simulink model "Top_Level"  (R2024b)
settings: Solver=ode3  StartTime=0.0  StopTime=1000  RelTol=1e-3  EnableMultiTasking=on
undefined symbols (not defined in the file): dspblkCoreblockFVToolHelper, gcbh, Theta1
libraries: arduinolib x4, arduinosensorlib x3, embeddedblockslib x2
settings Model: ExtModeTrigDuration=2  Creator=muham  LastModifiedBy=muham
settings SolverCC: AlgebraicLoopSolver=TrustRegion  AutoInsertRateTranBlk=on
settings DataIOCC: LimitDataPoints=on  SaveFormat=Array
settings OptimizationCC: ReuseModelBlockBuffer=off  ExpressionDepthLimit=2147483647  LifeSpan=Inf  MaxStackSize=64
settings DebuggingCC: UnderspecifiedInitializationDetection=Classic  MergeDetectMultiDrivingBlocksExec=none  FcnCallInpInsideContextMsg=warning  UnconnectedInputMsg=warning  UnconnectedOutputMsg=warning  UnconnectedLineMsg=warning  AllowSymbolicDim=off  StateNameClashWarn=warning  SFUnexpectedBacktrackingDiag=warning  SFNoUnconditionalDefaultTransitionDiag=warning  SFExecutionAtInitializationDiag=none  ArithmeticOperatorsInVariantConditions=warning
settings HardwareCC: ProdBitPerPointer=32  ProdBitPerSizeT=32  ProdBitPerPtrDiffT=32  ProdLargestAtomicInteger=Long  ProdLargestAtomicFloat=Double  ProdWordSize=32  ProdHWDeviceType=ARM Compatible->ARM Cortex
settings ModelReferenceCC: EnableRefExpFcnMdlSchedulingChecks=on  PropagateSignalLabelsOutOfModel=off
settings SFSimCC: SimUseLocalCustomCode=off  CustomCodeUndefinedFunction=UseInterfaceOnly  SimTargetLang=C++
settings RTWCC: Description=Embedded Coder  SystemTargetFile=ert.tlc  HardwareBoard=ESP32-WROOM(Arduino Compatible)  TemplateMakefile=ert_default_tmf  GenerateReport=on  RTWVerbose=off  RTWUseLocalCustomCode=off  Toolchain=ESP32  BuildConfiguration=Faster Runs  LaunchReport=on  CodeExecutionProfiling=on  GPUComputeCapability=3.5
settings CodeAppCC: ForceParamTrailComments=on  OperatorAnnotations=on  StateflowObjectComments=on  MATLABSourceComments=on
settings ERTTargetCC: TargetLangStandard=C99 (ISO)  MultiwordLength=2048  ERTCustomFileBanners=off  SupportContinuousTime=on  SupportNonInlinedSFcns=on  RemoveResetFunc=off  SupportVariableSizeSignals=on  ModelStepFunctionPrototypeControlCompliant=off  ExtModeTransport=3  ExtModeStaticAlloc=on  ExtModeAutomaticAllocSize=off  ExtModeStaticAllocSize=65536  ExtModeMexFile=ext_xcp  ExtModeIntrfLevel=Level2 - Open  InlinedParameterPlacement=Hierarchical  DynamicArrayContainerType=coder::array
settings ConfigComp: CovMetricSettings=dw  CovSaveCumulativeToWorkspaceVar=on  CovSaveSingleToWorkspaceVar=on  CovExternalEMLEnable=off  CovSFcnEnable=off

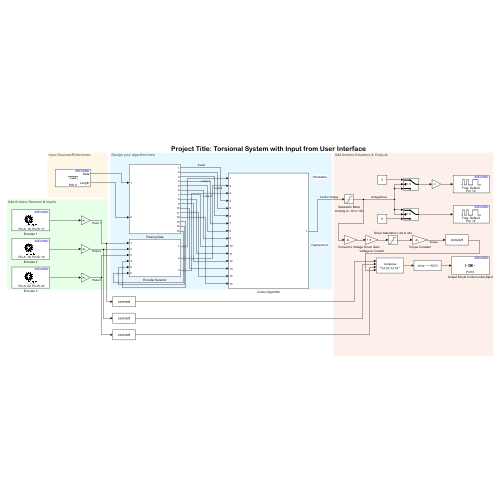
[thumbnail: Simulink's stored preview of the top-level diagram]
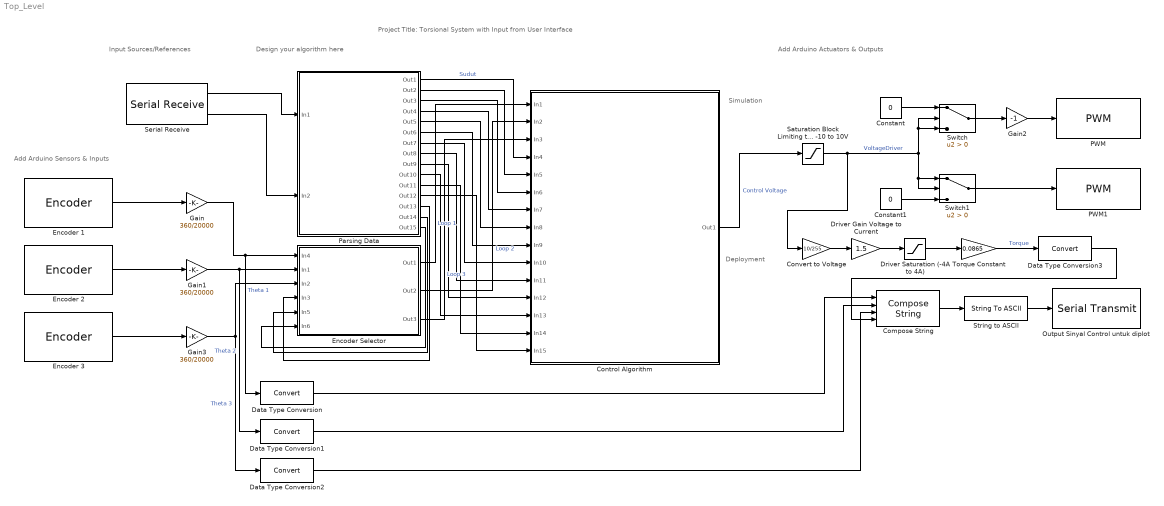
== system Top_Level ==
  note: Deployment
  note: Simulation
  note: Add Arduino Actuators & Outputs
  note: Add Arduino Sensors & Inputs
  note: Design your algorithm here
  note: Input Sources/References
  note: Project Title: Torsional System with Input from User Interface
  Compose String : ComposeString  Format="\"%f,%f,%f,%f\""
  Constant : Constant  Value=0  SampleTime=0.015
  Constant1 : Constant  Value=0  SampleTime=0.015
  Control Algorithm : Subsystem
  Convert to Voltage : Gain  Gain=10/255
  Data Type Conversion{,1..3} (4 alike) : DataTypeConversion  SaturateOnIntegerOverflow=off  RndMeth=Floor
  Driver Gain Voltage to Current : Gain  Gain=1.5
  Driver Saturation (-4A to 4A) : Saturate  UpperLimit=4  LowerLimit=-4
  Encoder 1 : arduinosensorlib/Encoder  InputA=16  InputB=17  Mode=No reset  SampleTime=0.015
  Encoder 2 : arduinosensorlib/Encoder  InputA=18  InputB=19  Mode=No reset  SampleTime=0.015
  Encoder 3 : arduinosensorlib/Encoder  InputA=22  InputB=23  Mode=No reset  SampleTime=0.015
  Encoder Selector : Subsystem
  Gain : Gain  Gain=360/20000
  Gain1 : Gain  Gain=360/20000
  Gain2 : Gain  Gain=-1
  Gain3 : Gain  Gain=360/20000
  Output Sinyal Control untuk diplot : arduinolib/Serial Transmit  portNumber=0  sendmode=write  label=Theta1:  sendformat=Decimal  floatprecision=4  header=uint8('(')  terminator=uint8(')')  blockPlatform=ARDUINO
  PWM : arduinolib/PWM  pinNumber=12  frequencyType=Default  desiredFrequency=490.2  achievableFrequency=490.2
  PWM1 : arduinolib/PWM  pinNumber=14  frequencyType=Default  desiredFrequency=490.2  achievableFrequency=490.2
  Parsing Data : Subsystem
  Saturation Block Limiting to -10 to 10V : Saturate  UpperLimit=255  LowerLimit=-255  OutDataTypeStr=int32
  Serial Receive : arduinolib/Serial Receive  portNumber=0  DataType=uint8  blockPlatform=ARDUINO  TimeOut=0  MaxDataLength=256  isARMArch=off  DataLengthOption=Variable length  Datalength=1  Header=[]  Terminator=[]  SampleTime=0.015  ShowOutStatus=on
  String to ASCII : StringToASCII  OutputVectorSize=48
  Switch : Switch  Criteria=u2 > Threshold  SaturateOnIntegerOverflow=off  InputSameDT=off
  Switch1 : Switch  Criteria=u2 > Threshold  SaturateOnIntegerOverflow=off  InputSameDT=off
  Torque Constant : Gain  Gain=0.0865
  wires:
  Encoder Selector/1(Out1) -> Control Algorithm/1(In1)  "Loop 1"
  Encoder Selector/2(Out2) -> Control Algorithm/2(In2)  "Loop 2"
  Encoder Selector/3(Out3) -> Control Algorithm/3(In3)  "Loop 3"
  Serial Receive/1 -> Parsing Data/1(In1)
  Serial Receive/2 -> Parsing Data/2(In2)
  Parsing Data/1(Out1) -> Control Algorithm/4(In4)  "Sudut"
  Parsing Data/2(Out2) -> Control Algorithm/5(In5)
  Encoder 1/1 -> Gain/1
  Encoder 2/1 -> Gain1/1
  Encoder 3/1 -> Gain3/1
  Parsing Data/13(Out13) -> Encoder Selector/4(In3)
  Parsing Data/14(Out14) -> Encoder Selector/5(In5)
  Parsing Data/15(Out15) -> Encoder Selector/6(In6)
  Parsing Data/3(Out3) -> Control Algorithm/6(In6)
  Parsing Data/4(Out4) -> Control Algorithm/7(In7)
  Parsing Data/5(Out5) -> Control Algorithm/8(In8)
  Parsing Data/6(Out6) -> Control Algorithm/9(In9)
  Parsing Data/7(Out7) -> Control Algorithm/10(In10)
  Parsing Data/8(Out8) -> Control Algorithm/11(In11)
  Parsing Data/9(Out9) -> Control Algorithm/12(In12)
  Parsing Data/10(Out10) -> Control Algorithm/13(In13)
  Parsing Data/11(Out11) -> Control Algorithm/14(In14)
  Parsing Data/12(Out12) -> Control Algorithm/15(In15)
  Saturation Block Limiting to -10 to 10V/1 -> Convert to Voltage/1, Switch1/2, Switch1/1, Switch/2, Switch/3  "VoltageDriver"
  Constant1/1 -> Switch1/3
  Control Algorithm/1(Out1) -> Saturation Block Limiting to -10 to 10V/1  "Control Voltage"
  Gain2/1 -> PWM/1
  Switch/1 -> Gain2/1
  Constant/1 -> Switch/1
  Switch1/1 -> PWM1/1
  Gain/1 -> Data Type Conversion/1, Encoder Selector/1(In4)  "Theta 1"
  Gain1/1 -> Data Type Conversion1/1, Encoder Selector/2(In1)  "Theta 2"
  Gain3/1 -> Data Type Conversion2/1, Encoder Selector/3(In2)  "Theta 3"
  Data Type Conversion/1 -> Compose String/1
  Driver Gain Voltage to Current/1 -> Driver Saturation (-4A to 4A)/1
  Driver Saturation (-4A to 4A)/1 -> Torque Constant/1
  Torque Constant/1 -> Data Type Conversion3/1  "Torque"
  Data Type Conversion1/1 -> Compose String/2
  Data Type Conversion2/1 -> Compose String/3
  Data Type Conversion3/1 -> Compose String/4
  String to ASCII/1 -> Output Sinyal Control untuk diplot/1
  Compose String/1 -> String to ASCII/1
  Convert to Voltage/1 -> Driver Gain Voltage to Current/1

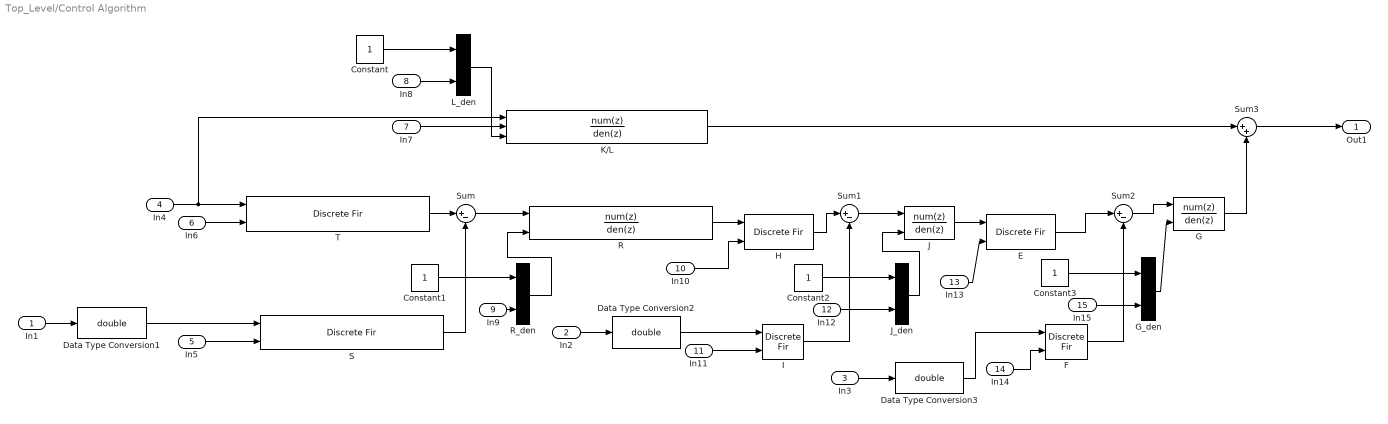
== system Top_Level/Control Algorithm ==
  In1 : Inport
  In2 : Inport  Port=2
  In3 : Inport  Port=3
  In4 : Inport  Port=4
  In5 : Inport  Port=5
  In6 : Inport  Port=6
  In7 : Inport  Port=7
  In8 : Inport  Port=8
  In9 : Inport  Port=9
  In10 : Inport  Port=10
  In11 : Inport  Port=11
  In12 : Inport  Port=12
  In13 : Inport  Port=13
  In14 : Inport  Port=14
  In15 : Inport  Port=15
  Constant{,1..3} (4 alike) : Constant  SampleTime=0.015
  Data Type Conversion1 : DataTypeConversion  OutDataTypeStr=double  SaturateOnIntegerOverflow=off  RndMeth=Floor
  Data Type Conversion2 : DataTypeConversion  OutDataTypeStr=double  SaturateOnIntegerOverflow=off  RndMeth=Floor
  Data Type Conversion3 : DataTypeConversion  OutDataTypeStr=double  SaturateOnIntegerOverflow=off  RndMeth=Floor
  E : DiscreteFir  LoadFcn=dspblkCoreblockFVToolHelper(gcbh,'load');  CoefSource=Input port  Coefficients=[1 1]
      settings: CopyFcn=dspblkCoreblockFVToolHelper(gcbh,'copy');  DeleteFcn=dspblkCoreblockFVToolHelper(gcbh,'close');  ModelCloseFcn=dspblkCoreblockFVToolHelper(gcbh,'close');  PreSaveFcn=dspblkCoreblockFVToolHelper(gcbh,'presave');  PostSaveFcn=dspblkCoreblockFVToolHelper(gcbh,'postsave');  CloseFcn=dspblkCoreblockFVToolHelper(gcbh,'close');  InputPortMap=u0,u1
  F : DiscreteFir  LoadFcn=dspblkCoreblockFVToolHelper(gcbh,'load');  CoefSource=Input port  Coefficients=[1 1]
      settings: CopyFcn=dspblkCoreblockFVToolHelper(gcbh,'copy');  DeleteFcn=dspblkCoreblockFVToolHelper(gcbh,'close');  ModelCloseFcn=dspblkCoreblockFVToolHelper(gcbh,'close');  PreSaveFcn=dspblkCoreblockFVToolHelper(gcbh,'presave');  PostSaveFcn=dspblkCoreblockFVToolHelper(gcbh,'postsave');  CloseFcn=dspblkCoreblockFVToolHelper(gcbh,'close');  InputPortMap=u0,u1
  G : DiscreteFilter  LoadFcn=dspblkCoreblockFVToolHelper(gcbh,'load');  DenominatorSource=Input port  Denominator=[1 1]  a0EqualsOne=on
      settings: CopyFcn=dspblkCoreblockFVToolHelper(gcbh,'copy');  DeleteFcn=dspblkCoreblockFVToolHelper(gcbh,'close');  ModelCloseFcn=dspblkCoreblockFVToolHelper(gcbh,'close');  PreSaveFcn=dspblkCoreblockFVToolHelper(gcbh,'presave');  PostSaveFcn=dspblkCoreblockFVToolHelper(gcbh,'postsave');  CloseFcn=dspblkCoreblockFVToolHelper(gcbh,'close');  InputPortMap=u0,p3
  G_den : Mux  Inputs=2
  H : DiscreteFir  LoadFcn=dspblkCoreblockFVToolHelper(gcbh,'load');  CoefSource=Input port  Coefficients=[1 1]
      settings: CopyFcn=dspblkCoreblockFVToolHelper(gcbh,'copy');  DeleteFcn=dspblkCoreblockFVToolHelper(gcbh,'close');  ModelCloseFcn=dspblkCoreblockFVToolHelper(gcbh,'close');  PreSaveFcn=dspblkCoreblockFVToolHelper(gcbh,'presave');  PostSaveFcn=dspblkCoreblockFVToolHelper(gcbh,'postsave');  CloseFcn=dspblkCoreblockFVToolHelper(gcbh,'close');  InputPortMap=u0,u1
  I : DiscreteFir  LoadFcn=dspblkCoreblockFVToolHelper(gcbh,'load');  CoefSource=Input port  Coefficients=[1 1]
      settings: CopyFcn=dspblkCoreblockFVToolHelper(gcbh,'copy');  DeleteFcn=dspblkCoreblockFVToolHelper(gcbh,'close');  ModelCloseFcn=dspblkCoreblockFVToolHelper(gcbh,'close');  PreSaveFcn=dspblkCoreblockFVToolHelper(gcbh,'presave');  PostSaveFcn=dspblkCoreblockFVToolHelper(gcbh,'postsave');  CloseFcn=dspblkCoreblockFVToolHelper(gcbh,'close');  InputPortMap=u0,u1
  J : DiscreteFilter  LoadFcn=dspblkCoreblockFVToolHelper(gcbh,'load');  DenominatorSource=Input port  Denominator=[1 1]  a0EqualsOne=on
      settings: CopyFcn=dspblkCoreblockFVToolHelper(gcbh,'copy');  DeleteFcn=dspblkCoreblockFVToolHelper(gcbh,'close');  ModelCloseFcn=dspblkCoreblockFVToolHelper(gcbh,'close');  PreSaveFcn=dspblkCoreblockFVToolHelper(gcbh,'presave');  PostSaveFcn=dspblkCoreblockFVToolHelper(gcbh,'postsave');  CloseFcn=dspblkCoreblockFVToolHelper(gcbh,'close');  InputPortMap=u0,p3
  J_den : Mux  Inputs=2
  K/L : DiscreteFilter  LoadFcn=dspblkCoreblockFVToolHelper(gcbh,'load');  NumeratorSource=Input port  Numerator=[1 1 1 1 1 1 1 1]  DenominatorSource=Input port  Denominator=[1 1 1 1 1 1 1 1]  a0EqualsOne=on
      settings: CopyFcn=dspblkCoreblockFVToolHelper(gcbh,'copy');  DeleteFcn=dspblkCoreblockFVToolHelper(gcbh,'close');  ModelCloseFcn=dspblkCoreblockFVToolHelper(gcbh,'close');  PreSaveFcn=dspblkCoreblockFVToolHelper(gcbh,'presave');  PostSaveFcn=dspblkCoreblockFVToolHelper(gcbh,'postsave');  CloseFcn=dspblkCoreblockFVToolHelper(gcbh,'close');  InputPortMap=u0,p1,p3
  L_den : Mux  Inputs=2
  R : DiscreteFilter  LoadFcn=dspblkCoreblockFVToolHelper(gcbh,'load');  DenominatorSource=Input port  Denominator=[1 1 1 1 1 1 1 1]  a0EqualsOne=on
      settings: CopyFcn=dspblkCoreblockFVToolHelper(gcbh,'copy');  DeleteFcn=dspblkCoreblockFVToolHelper(gcbh,'close');  ModelCloseFcn=dspblkCoreblockFVToolHelper(gcbh,'close');  PreSaveFcn=dspblkCoreblockFVToolHelper(gcbh,'presave');  PostSaveFcn=dspblkCoreblockFVToolHelper(gcbh,'postsave');  CloseFcn=dspblkCoreblockFVToolHelper(gcbh,'close');  InputPortMap=u0,p3
  R_den : Mux  Inputs=2
  S : DiscreteFir  LoadFcn=dspblkCoreblockFVToolHelper(gcbh,'load');  CoefSource=Input port  Coefficients=[1 1 1 1 1 1 1 1]
      settings: CopyFcn=dspblkCoreblockFVToolHelper(gcbh,'copy');  DeleteFcn=dspblkCoreblockFVToolHelper(gcbh,'close');  ModelCloseFcn=dspblkCoreblockFVToolHelper(gcbh,'close');  PreSaveFcn=dspblkCoreblockFVToolHelper(gcbh,'presave');  PostSaveFcn=dspblkCoreblockFVToolHelper(gcbh,'postsave');  CloseFcn=dspblkCoreblockFVToolHelper(gcbh,'close');  InputPortMap=u0,u1
  Sum : Sum  Inputs=|+-
  Sum1 : Sum  Inputs=|+-
  Sum2 : Sum  Inputs=|+-
  Sum3 : Sum  Inputs=|++
  T : DiscreteFir  LoadFcn=dspblkCoreblockFVToolHelper(gcbh,'load');  CoefSource=Input port  Coefficients=[1 1 1 1 1 1 1 1]
      settings: CopyFcn=dspblkCoreblockFVToolHelper(gcbh,'copy');  DeleteFcn=dspblkCoreblockFVToolHelper(gcbh,'close');  ModelCloseFcn=dspblkCoreblockFVToolHelper(gcbh,'close');  PreSaveFcn=dspblkCoreblockFVToolHelper(gcbh,'presave');  PostSaveFcn=dspblkCoreblockFVToolHelper(gcbh,'postsave');  CloseFcn=dspblkCoreblockFVToolHelper(gcbh,'close');  InputPortMap=u0,u1
  Out1 : Outport
  wires:
  In1/1 -> Data Type Conversion1/1
  T/1 -> Sum/1
  S/1 -> Sum/2
  Sum/1 -> R/1
  In4/1 -> K/L/1, T/1
  R/1 -> H/1
  In2/1 -> Data Type Conversion2/1
  I/1 -> Sum1/2
  H/1 -> Sum1/1
  Sum1/1 -> J/1
  J/1 -> E/1
  In3/1 -> Data Type Conversion3/1
  E/1 -> Sum2/1
  F/1 -> Sum2/2
  Sum2/1 -> G/1
  K/L/1 -> Sum3/1
  G/1 -> Sum3/2
  In5/1 -> S/2
  In6/1 -> T/2
  In7/1 -> K/L/2
  L_den/1 -> K/L/3
  In8/1 -> L_den/2
  Constant/1 -> L_den/1
  Constant1/1 -> R_den/1
  In9/1 -> R_den/2
  R_den/1 -> R/2
  In10/1 -> H/2
  In11/1 -> I/2
  J_den/1 -> J/2
  Constant2/1 -> J_den/1
  In12/1 -> J_den/2
  In13/1 -> E/2
  In14/1 -> F/2
  Constant3/1 -> G_den/1
  In15/1 -> G_den/2
  G_den/1 -> G/2
  Data Type Conversion1/1 -> S/1
  Data Type Conversion2/1 -> I/1
  Data Type Conversion3/1 -> F/1
  Sum3/1 -> Out1/1

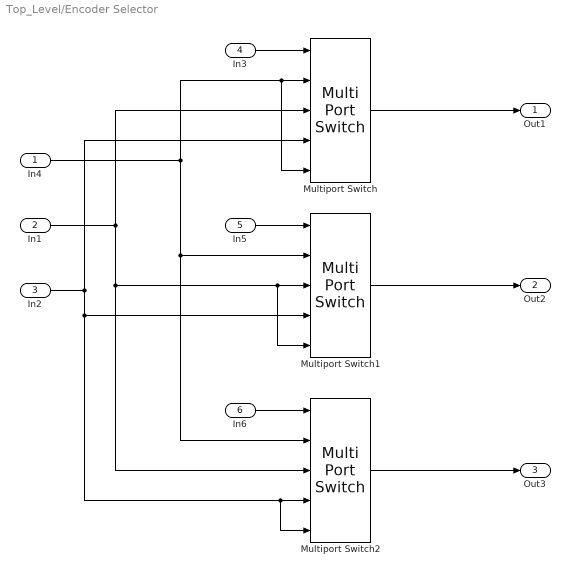
== system Top_Level/Encoder Selector ==
  In4 : Inport
  In1 : Inport  Port=2
  In2 : Inport  Port=3
  In3 : Inport  Port=4
  In5 : Inport  Port=5
  In6 : Inport  Port=6
  Multiport Switch : MultiPortSwitch  DataPortForDefault=Additional data port  DiagnosticForDefault=None  SaturateOnIntegerOverflow=off  InputSameDT=off
  Multiport Switch1 : MultiPortSwitch  DataPortForDefault=Additional data port  DiagnosticForDefault=None  SaturateOnIntegerOverflow=off  InputSameDT=off
  Multiport Switch2 : MultiPortSwitch  DataPortForDefault=Additional data port  DiagnosticForDefault=None  SaturateOnIntegerOverflow=off  InputSameDT=off
  Out1 : Outport
  Out2 : Outport  Port=2
  Out3 : Outport  Port=3
  wires:
  Multiport Switch/1 -> Out1/1
  Multiport Switch1/1 -> Out2/1
  Multiport Switch2/1 -> Out3/1
  In4/1 -> Multiport Switch2/2, Multiport Switch1/2, Multiport Switch/5, Multiport Switch/2
  In1/1 -> Multiport Switch2/3, Multiport Switch1/5, Multiport Switch1/3, Multiport Switch/3
  In2/1 -> Multiport Switch2/5, Multiport Switch2/4, Multiport Switch1/4, Multiport Switch/4
  In3/1 -> Multiport Switch/1
  In5/1 -> Multiport Switch1/1
  In6/1 -> Multiport Switch2/1

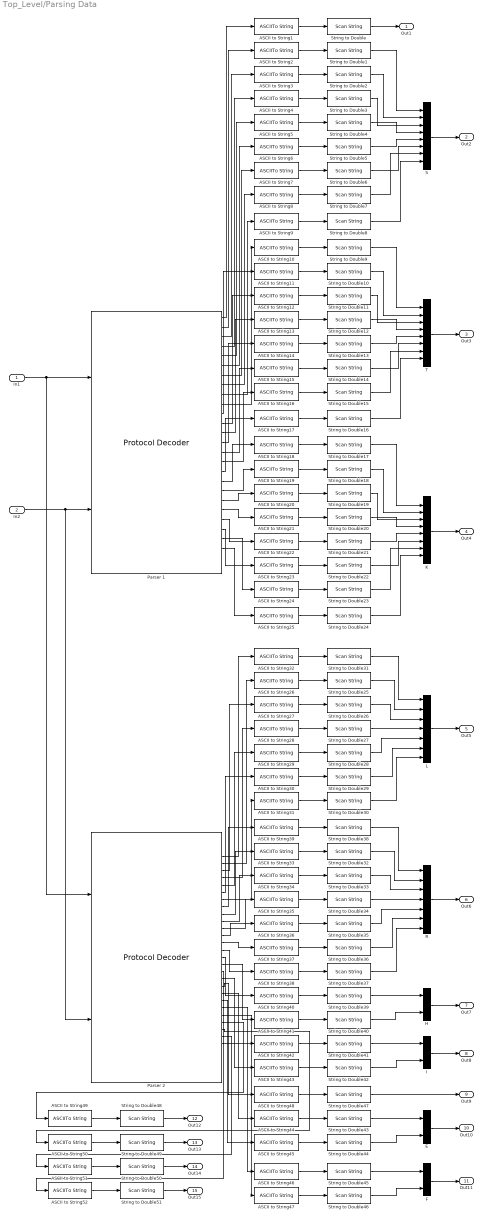
== system Top_Level/Parsing Data ==
  In1 : Inport
  In2 : Inport  Port=2
  ASCII to String{1..52} (52 alike) : ASCIIToString
  E : Mux  Inputs=2
  F : Mux  Inputs=2
  H : Mux  Inputs=2
  I : Mux  Inputs=2
  K : Mux  Inputs=8
  L : Mux  Inputs=7
  Parser 1 : embeddedblockslib/Protocol Decoder  IsParseCSV=on  Header=uint8('#')  FieldTable={ 'Sudut', '4', 'uint8', 'Little endian'; 'S0', '6', 'uint8', 'Little endian'; 'S1', '6', 'uint8', 'Little endian'; 'S2', '6', 'uint8', 'Little endian'; 'S3', '6', 'uint8', 'Little endian'; 'S4', '6', 'uint8', 'Little endian'; 'S5', '6', 'uint8', 'Little endian'; 'S6', '6', 'uint8', 'Little endian'; 'S7', '6', 'uint8', 'Little endian'; 'T0', '6', 'uint8', 'Little endian'; 'T1', '6', 'uint8', 'Little endian'; 'T2', '6', 'uint8', 'Little endian'; 'T3', '6', 'uint8', 'Little endian'; 'T4', '6', 'uint8', 'Little endian'; 'T5', '6', 'uint8', 'Little endian'; 'T6', '6', 'uint8', 'Little endian'; 'T7', '6', 'uint8', 'Little endian'; 'K0', '6', 'uint8', 'Little endian'; 'K1', '6', 'uint8', 'Little endian'; 'K2', '6', 'uint8', 'Little endian'; 'K3', '6', 'uint8', 'Little endian'; 'K4', '6', 'uint8', 'Little endian'; 'K5', '6', 'uint8', 'Little endian'; 'K6', '6', 'uint8', 'Little endian'; 'K7', '6', 'uint8', 'Little endian' }  IsVariableSizeLastField=off  MaxVariableSizeFieldLength=[]  IsChecksumRequired=off  ChecksumAlgorithm=XOR of bytes  ChecksumSize=[]  TerminatorOption=Custom terminator  CustomTerminatorVal=uint8('$')  IsInputLengthAvailable=on  Logo=ARDUINO
      settings: LibrarySourceBlock=arduinolib/Protocol Decoder
  Parser 2 : embeddedblockslib/Protocol Decoder  IsParseCSV=on  Header=uint8('%')  FieldTable={ 'L1', '6', 'uint8', 'Little endian'; 'L2', '6', 'uint8', 'Little endian'; 'L3', '6', 'uint8', 'Little endian'; 'L4', '6', 'uint8', 'Little endian'; 'L5', '6', 'uint8', 'Little endian'; 'L6', '6', 'uint8', 'Little endian'; 'L7', '6', 'uint8', 'Little endian'; 'R1', '6', 'uint8', 'Little endian'; 'R2', '6', 'uint8', 'Little endian'; 'R3', '6', 'uint8', 'Little endian'; 'R4', '6', 'uint8', 'Little endian'; 'R5', '6', 'uint8', 'Little endian'; 'R6', '6', 'uint8', 'Little endian'; 'R7', '6', 'uint8', 'Little endian'; 'H0', '6', 'uint8', 'Little endian'; 'H1', '6', 'uint8', 'Little endian'; 'I0', '6', 'uint8', 'Little endian'; 'I1', '6', 'uint8', 'Little endian'; 'J1', '6', 'uint8', 'Little endian'; 'E0', '6', 'uint8', 'Little endian'; 'E1', '6', 'uint8', 'Little endian'; 'F0', '6', 'uint8', 'Little endian'; 'F1', '6', 'uint8', 'Little endian'; 'G1', '6', 'uint8', 'Little endian'; 'enc1', '1', 'uint8', 'Little endian'; 'enc2', '1', 'uint8', 'Little endian'; 'enc3', '1', 'uint8', 'Little endian' }  IsVariableSizeLastField=off  MaxVariableSizeFieldLength=[]  IsChecksumRequired=off  ChecksumAlgorithm=XOR of bytes  ChecksumSize=[]  TerminatorOption=Custom terminator  CustomTerminatorVal=uint8('^')  IsInputLengthAvailable=on  Logo=ARDUINO
      settings: LibrarySourceBlock=arduinolib/Protocol Decoder
  R : Mux  Inputs=7
  S : Mux  Inputs=8
  String to Double{,1..51} (52 alike) : ScanString  Format="\"%lf\""
  T : Mux  Inputs=8
  Out1 : Outport
  Out2 : Outport  Port=2
  Out3 : Outport  Port=3
  Out4 : Outport  Port=4
  Out5 : Outport  Port=5
  Out6 : Outport  Port=6
  Out7 : Outport  Port=7
  Out8 : Outport  Port=8
  Out9 : Outport  Port=9
  Out10 : Outport  Port=10
  Out11 : Outport  Port=11
  Out12 : Outport  Port=12
  Out13 : Outport  Port=13
  Out14 : Outport  Port=14
  Out15 : Outport  Port=15
  wires:
  In1/1 -> Parser 2/1, Parser 1/1
  In2/1 -> Parser 2/2, Parser 1/2
  ASCII to String1/1 -> String to Double/1
  String to Double/1 -> Out1/1
  Parser 1/1 -> ASCII to String1/1
  Parser 1/2 -> ASCII to String2/1
  ASCII to String2/1 -> String to Double1/1
  ASCII to String3/1 -> String to Double2/1
  Parser 1/3 -> ASCII to String3/1
  ASCII to String5/1 -> String to Double4/1
  ASCII to String4/1 -> String to Double3/1
  ASCII to String6/1 -> String to Double5/1
  Parser 1/4 -> ASCII to String4/1
  Parser 1/5 -> ASCII to String5/1
  Parser 1/6 -> ASCII to String6/1
  ASCII to String8/1 -> String to Double7/1
  ASCII to String7/1 -> String to Double6/1
  Parser 1/7 -> ASCII to String7/1
  Parser 1/8 -> ASCII to String8/1
  ASCII to String9/1 -> String to Double8/1
  Parser 1/9 -> ASCII to String9/1
  String to Double1/1 -> S/1
  String to Double2/1 -> S/2
  String to Double3/1 -> S/3
  String to Double4/1 -> S/4
  String to Double5/1 -> S/5
  String to Double6/1 -> S/6
  String to Double7/1 -> S/7
  String to Double8/1 -> S/8
  S/1 -> Out2/1
  ASCII to String10/1 -> String to Double9/1
  ASCII to String15/1 -> String to Double14/1
  ASCII to String16/1 -> String to Double15/1
  ASCII to String11/1 -> String to Double10/1
  T/1 -> Out3/1
  String to Double15/1 -> T/7
  String to Double14/1 -> T/6
  String to Double12/1 -> T/4
  ASCII to String12/1 -> String to Double11/1
  ASCII to String13/1 -> String to Double12/1
  String to Double10/1 -> T/2
  String to Double9/1 -> T/1
  String to Double11/1 -> T/3
  ASCII to String14/1 -> String to Double13/1
  String to Double16/1 -> T/8
  ASCII to String17/1 -> String to Double16/1
  String to Double13/1 -> T/5
  Parser 1/10 -> ASCII to String10/1
  Parser 1/11 -> ASCII to String11/1
  Parser 1/13 -> ASCII to String13/1
  Parser 1/14 -> ASCII to String14/1
  Parser 1/15 -> ASCII to String15/1
  Parser 1/16 -> ASCII to String16/1
  Parser 1/17 -> ASCII to String17/1
  Parser 1/12 -> ASCII to String12/1
  ASCII to String18/1 -> String to Double17/1
  ASCII to String23/1 -> String to Double22/1
  ASCII to String24/1 -> String to Double23/1
  ASCII to String19/1 -> String to Double18/1
  K/1 -> Out4/1
  String to Double23/1 -> K/7
  String to Double22/1 -> K/6
  String to Double20/1 -> K/4
  ASCII to String20/1 -> String to Double19/1
  ASCII to String21/1 -> String to Double20/1
  String to Double18/1 -> K/2
  String to Double17/1 -> K/1
  String to Double19/1 -> K/3
  ASCII to String22/1 -> String to Double21/1
  String to Double24/1 -> K/8
  ASCII to String25/1 -> String to Double24/1
  String to Double21/1 -> K/5
  Parser 1/18 -> ASCII to String18/1
  Parser 1/19 -> ASCII to String19/1
  Parser 1/20 -> ASCII to String20/1
  Parser 1/21 -> ASCII to String21/1
  Parser 1/22 -> ASCII to String22/1
  Parser 1/23 -> ASCII to String23/1
  Parser 1/24 -> ASCII to String24/1
  Parser 1/25 -> ASCII to String25/1
  ASCII to String26/1 -> String to Double25/1
  ASCII to String27/1 -> String to Double26/1
  String to Double31/1 -> L/1
  String to Double27/1 -> L/4
  String to Double29/1 -> L/6
  ASCII to String29/1 -> String to Double28/1
  ASCII to String31/1 -> String to Double30/1
  ASCII to String32/1 -> String to Double31/1
  String to Double26/1 -> L/3
  String to Double25/1 -> L/2
  ASCII to String30/1 -> String to Double29/1
  L/1 -> Out5/1
  String to Double30/1 -> L/7
  ASCII to String28/1 -> String to Double27/1
  Parser 2/1 -> ASCII to String32/1
  Parser 2/2 -> ASCII to String26/1
  Parser 2/3 -> ASCII to String27/1
  Parser 2/4 -> ASCII to String28/1
  Parser 2/5 -> ASCII to String29/1
  Parser 2/6 -> ASCII to String30/1
  Parser 2/7 -> ASCII to String31/1
  String to Double28/1 -> L/5
  ASCII to String35/1 -> String to Double34/1
  String to Double32/1 -> R/2
  R/1 -> Out6/1
  ASCII to String37/1 -> String to Double36/1
  ASCII to String36/1 -> String to Double35/1
  String to Double33/1 -> R/3
  ASCII to String38/1 -> String to Double37/1
  String to Double37/1 -> R/7
  ASCII to String33/1 -> String to Double32/1
  String to Double38/1 -> R/1
  String to Double36/1 -> R/6
  String to Double34/1 -> R/4
  String to Double35/1 -> R/5
  ASCII to String34/1 -> String to Double33/1
  Parser 2/8 -> ASCII to String39/1
  Parser 2/9 -> ASCII to String33/1
  Parser 2/10 -> ASCII to String34/1
  Parser 2/11 -> ASCII to String35/1
  Parser 2/12 -> ASCII to String36/1
  Parser 2/13 -> ASCII to String37/1
  Parser 2/14 -> ASCII to String38/1
  ASCII to String40/1 -> String to Double39/1
  ASCII to String41/1 -> String to Double40/1
  H/1 -> Out7/1
  String to Double40/1 -> H/2
  String to Double39/1 -> H/1
  Parser 2/15 -> ASCII to String40/1
  Parser 2/16 -> ASCII to String41/1
  ASCII to String43/1 -> String to Double42/1
  String to Double41/1 -> I/1
  ASCII to String42/1 -> String to Double41/1
  I/1 -> Out8/1
  String to Double42/1 -> I/2
  Parser 2/17 -> ASCII to String42/1
  Parser 2/18 -> ASCII to String43/1
  ASCII to String44/1 -> String to Double43/1
  String to Double44/1 -> E/2
  String to Double43/1 -> E/1
  ASCII to String45/1 -> String to Double44/1
  E/1 -> Out10/1
  Parser 2/20 -> ASCII to String44/1
  Parser 2/21 -> ASCII to String45/1
  ASCII to String46/1 -> String to Double45/1
  F/1 -> Out11/1
  ASCII to String47/1 -> String to Double46/1
  String to Double46/1 -> F/2
  String to Double45/1 -> F/1
  Parser 2/22 -> ASCII to String46/1
  Parser 2/23 -> ASCII to String47/1
  Parser 2/24 -> ASCII to String49/1
  Parser 2/25 -> ASCII to String50/1
  Parser 2/26 -> ASCII to String51/1
  Parser 2/27 -> ASCII to String52/1
  String to Double47/1 -> Out9/1
  Parser 2/19 -> ASCII to String48/1
  ASCII to String48/1 -> String to Double47/1
  ASCII to String49/1 -> String to Double48/1
  String to Double48/1 -> Out12/1
  ASCII to String50/1 -> String to Double49/1
  String to Double49/1 -> Out13/1
  ASCII to String51/1 -> String to Double50/1
  String to Double50/1 -> Out14/1
  ASCII to String52/1 -> String to Double51/1
  String to Double51/1 -> Out15/1
  ASCII to String39/1 -> String to Double38/1
